simulink model "Trim_Model"  (R2012b)
settings: Solver=ode23tb  StartTime=0.0  StopTime=inf  FixedStep=0.001  MaxStep=0.01  RelTol=1e-5
values from neighbouring files (symbols this model uses):
  a = 2.1117    [SetupComplete.m]
  A_x = 0.015    [SetupComplete.m]
  A_y = A_x    (= 0.015)    [SetupComplete.m]
  A_z = 0.16    [SetupComplete.m]
  C_d0 = 0.00209    [SetupComplete.m]
  C_x = 1.2    [SetupComplete.m]
  C_y = C_x    (= 1.2)    [SetupComplete.m]
  C_z = 2.2    [SetupComplete.m]
  CG_0 = [0,0,0.02]'    [SetupComplete.m]
  h = 0.08    [SetupComplete.m]
  h_FA = 0.02    [SetupComplete.m]
  h_M = 0.064    [SetupComplete.m]
  I_BAC_0 = [ Ix,0,Ixz;0,Iy,0;Ixz,0,Iz]    [SetupComplete.m]
  I_prop = 1/4*M_eq*R^2*diag([1,1,2])    [SetupComplete.m]
  I_tube = [1/2*M_tube*R_tube_eq^2,0,  0  ;           0 ,1/3*M_tube*l_arm^2,0;             0  ,0,1/3*M_tube*l_arm^2]    [SetupComplete.m]
  Initial_Omegas = [1;1;1]*Omega_hover    [Run3Copter.m]
  Initial_Torques = [1;1;1]*Torque_hover    [Run3Copter.m]
  J_FA = I_prop(1,1) + m_prop*h^2  + m_FA*h_FA^2 + m_M*h_M^2    [SetupComplete.m]
  J_T = J_m+1/2*M_eq*R^2    (= 2.000642e-05)    [SetupComplete.m]
  l = 0.345    [SetupComplete.m]
  l_arm = 0.264    [SetupComplete.m]
  m = 3.51    [SetupComplete.m]
  m_0 = 2.61    [SetupComplete.m]
  m_FA = 0.02    [SetupComplete.m]
  m_M = 0.300    (= 0.3)    [SetupComplete.m]
  m_prop = 0.02    [SetupComplete.m]
  Omega_hover = 570    [SetupComplete.m]
  R = 0.1778    [SetupComplete.m]
  rho = 1.15    [SetupComplete.m]
  Rotation_sign = [ 1,-1,-1]    [SetupComplete.m]
  sigma = b*c/(pi*R)    (= 0.107416159567)    [SetupComplete.m]
  Tau_motors = 0.06    [SetupComplete.m]
  theta_0 = 0.38397    [SetupComplete.m]
  theta_1 = -0.2967    [SetupComplete.m]
  Throttle_Hover = X(1)/16    [SetupComplete.m]
  v_i0 = sqrt( 1/3*m*g/(2*rho*pi*R^2)  )    [SetupComplete.m]
undefined symbols (not defined in the file or in its folder): Omega_TTO, Throtle_TTO, Torque_TTO, v_i_adim, Vx_adim, Vz_adim
libraries: vrlib x15, dspmtrx3 x11, simulink_extras x4, aerolibtransform2 x1
(part 2 of 2)

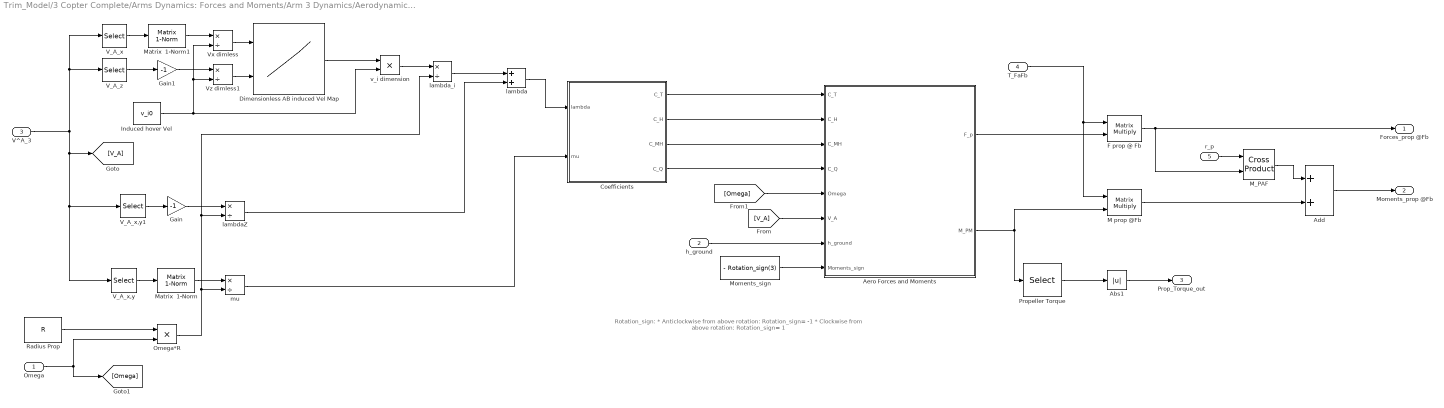
== system Trim_Model/3 Copter Complete/Arms Dynamics: Forces and Moments/Arm 3 Dynamics/Aerodynamics Propeller ==
  note: Rotation_sign:
      |
      | * Anticlockwise from above rotation: Rotation_sign= -1
      | * Clockwise from above rotation: Rotation_sign= 1
  Omega : Inport
  h_ground : Inport  Port=2
  "V^A_3 " : Inport  Port=3
  T_FaFb : Inport  Port=4
  r_p : Inport  Port=5
  Abs1 : Abs
  Add : Sum
  Aero Forces and Moments : MATLAB Function  TreatAsAtomicUnit=on
  Coefficients : MATLAB Function  TreatAsAtomicUnit=on
  Dimensionless AB induced Vel Map : Lookup_n-D  BreakpointsForDimension1=Vx_adim  BreakpointsForDimension2=Vz_adim  BreakpointsForDimension3=[5, 7]  Table=v_i_adim  RndMeth=Simplest  InputSameDT=on
  F prop @ Fb : Product  Multiplication=Matrix(*)
  Gain : Gain  Gain=-1
  Gain1 : Gain  Gain=-1
  Induced hover Vel : Constant  Value=v_i0
  M prop @Fb : Product  Multiplication=Matrix(*)
  M_PAF : vrlib/Utilities/Cross Product
  Matrix  1-Norm : dspmtrx3/Matrix  1-Norm  outputDataTypeStr=Inherit: Same as accumulator  outputLastDataTypeStr=Inherit: Same as accumulator  outputMin=[]  outputMax=[]  roundingMode=Floor  overflowMode=off
  Matrix  1-Norm1 : dspmtrx3/Matrix  1-Norm  outputDataTypeStr=Inherit: Same as accumulator  outputLastDataTypeStr=Inherit: Same as accumulator  outputMin=[]  outputMax=[]  roundingMode=Floor  overflowMode=off
  Moments_sign : Constant  Value=- Rotation_sign(3)
  Omega*R : Product  Inputs=**
  Propeller Torque : Selector  InputPortWidth=3  IndexOptions=Index vector (dialog)  Indices=3  OutputSizes=1
  Radius Prop : Constant  Value=R
  V_A_x : Selector  InputPortWidth=3  IndexOptions=Index vector (dialog)  Indices=[1 2]  OutputSizes=1
  V_A_x,y : Selector  InputPortWidth=3  IndexOptions=Index vector (dialog)  Indices=[1 2]  OutputSizes=1
  V_A_x,y1 : Selector  InputPortWidth=3  IndexOptions=Index vector (dialog)  Indices=[3]  OutputSizes=1
  V_A_z : Selector  InputPortWidth=3  IndexOptions=Index vector (dialog)  Indices=3  OutputSizes=1
  Vx dimless : Product  Inputs=*/
  Vz dimless1 : Product  Inputs=*/
  lambda : Sum
  lambdaZ : Product  Inputs=*/
  lambda_i : Product  Inputs=*/
  mu : Product  Inputs=*/
  v_i dimension : Product  Inputs=**
  Forces_prop @Fb : Outport
  Moments_prop @Fb : Outport  Port=2
  Prop_Torque_out : Outport  Port=3
  wires:
  Radius Prop/1 -> Omega*R/1
  Omega/1 -> Omega*R/2, [Omega]
  V_A_x,y/1 -> Matrix  1-Norm/1
  Matrix  1-Norm/1 -> mu/1
  Omega*R/1 -> mu/2, lambdaZ/2, lambda_i/2
  Vx dimless/1 -> Dimensionless AB induced Vel Map/1
  Vz dimless1/1 -> Dimensionless AB induced Vel Map/2
  Dimensionless AB induced Vel Map/1 -> v_i dimension/1
  v_i dimension/1 -> lambda_i/1
  V_A_x,y1/1 -> Gain/1
  Gain/1 -> lambdaZ/1
  lambda_i/1 -> lambda/1
  lambdaZ/1 -> lambda/2
  lambda/1 -> Coefficients/1(lambda)
  mu/1 -> Coefficients/2(mu)
  Coefficients/1(C_T) -> Aero Forces and Moments/1(C_T)
  Coefficients/2(C_H) -> Aero Forces and Moments/2(C_H)
  Coefficients/3(C_MH) -> Aero Forces and Moments/3(C_MH)
  Coefficients/4(C_Q) -> Aero Forces and Moments/4(C_Q)
  [V_A] -> Aero Forces and Moments/6(V_A)
  [Omega] -> Aero Forces and Moments/5(Omega)
  Aero Forces and Moments/2(M_PM) -> Propeller Torque/1, M prop @Fb/2
  Add/1 -> Moments_prop @Fb/1
  h_ground/1 -> Aero Forces and Moments/7(h_ground)
  Moments_sign/1 -> Aero Forces and Moments/8(Moments_sign)
  Propeller Torque/1 -> Abs1/1
  T_FaFb/1 -> M prop @Fb/1, F prop @ Fb/1
  Aero Forces and Moments/1(F_p) -> F prop @ Fb/2
  F prop @ Fb/1 -> M_PAF/2, Forces_prop @Fb/1
  r_p/1 -> M_PAF/1
  M_PAF/1 -> Add/1
  M prop @Fb/1 -> Add/2
  Abs1/1 -> Prop_Torque_out/1
  "V^A_3 "/1 -> [V_A], V_A_x,y1/1, V_A_x,y/1, V_A_z/1, V_A_x/1
  V_A_x/1 -> Matrix  1-Norm1/1
  V_A_z/1 -> Gain1/1
  Induced hover Vel/1 -> Vz dimless1/2, Vx dimless/2, v_i dimension/2
  Gain1/1 -> Vz dimless1/1
  Matrix  1-Norm1/1 -> Vx dimless/1

== system Trim_Model/3 Copter Complete/Arms Dynamics: Forces and Moments/Arm 3 Dynamics/Arms Kinematics ==
  note: Input angles in rads
      |
      | 1. eta_3 (rad)  (Pan arm 3)
      | 2. gamma_3 (rad)  (Tilt arm 3)
  Angles (rad) : Inport
  Angles_dot (rad/s) : Inport  Port=2
  Add : Sum
  Add3 : Sum
  Bus Creator : BusCreator  Inputs=2
  Cross Product : vrlib/Utilities/Cross Product
  DCM Arm 3 : MATLAB Function  TreatAsAtomicUnit=on
  Demux : Demux  Outputs=2
  Demux3 : Demux  Outputs=2
  Fa->Fb : Product  Multiplication=Matrix(*)
  Gain6 : Gain  Gain=[0;1;0]
  Gain7 : Gain  Gain=[0;0;-1]
  Gain8 : Gain  Gain=[-1/2;-sqrt(3)/2;0]
  Gain9 : Gain  Gain=[1;0;0]
  Matrix Multiply : Product  Multiplication=Matrix(*)
  Transpose : dspmtrx3/Transpose  Hermitian=off  overflowFlag=off
  h arm : Constant  Value=h
  length arm : Constant  Value=l
  r_p3 (m) : Outport
  r_p3_dot (m/s) : Outport  Port=2
  Arm DCMs : Outport  Port=3
  omega^3_Ab (rad/s) : Outport  Port=4
  wires:
  DCM Arm 3/1(T_Fb_FA) -> Transpose/1, Bus Creator/1  "T^3_Fb,FA"
  Bus Creator/1 -> Arm DCMs/1
  Transpose/1 -> [T3_F_aFb], Bus Creator/2  "T^3_F_a,Fb"
  Angles (rad)/1 -> Demux/1
  Demux/1 -> DCM Arm 3/1(eta_3)
  Demux/2 -> DCM Arm 3/2(gamma_3)
  Angles_dot (rad/s)/1 -> Demux3/1
  Demux3/2 -> Gain9/1  "gamma_dot_3"
  Demux3/1 -> Gain6/1  "eta_dot_3"
  Gain9/1 -> Matrix Multiply/2
  [T3_F_aFb] -> Matrix Multiply/1
  Matrix Multiply/1 -> Add/2
  Gain6/1 -> Add/1
  Add/1 -> Cross Product/1, omega^3_Ab (rad/s)/1  "omega^3_Ab"
  Add3/1 -> r_p3 (m)/1  "r_p3 (m)"
  length arm/1 -> Gain8/1
  h arm/1 -> Gain7/1
  Gain7/1 -> Fa->Fb/2
  [T3_F_aFb] -> Fa->Fb/1
  Gain8/1 -> Add3/1
  Fa->Fb/1 -> Cross Product/2, Add3/2
  Cross Product/1 -> r_p3_dot (m/s)/1

== system Trim_Model/3 Copter Complete/Arms Dynamics: Forces and Moments/Arm 3 Dynamics/ESC-MOTOR dynamics1 ==
  note: 1) Only subsystems can be added as variant choices at this level
      | 2) Blocks cannot be connected at this level as connectivity is
      | automatically determined at simulation, based on the active variant
  Throttle : Inport
  Omega : Inport  Port=2
  Initial Omega : Inport  Port=3
  Prop Torque : Inport  Port=4
  ESC+Motor Dynamcis COMPLETED : Subsystem  TreatAsAtomicUnit=on  VariantObject=Variant_completed
  ESC+Motor Dynamcis SYMPLIFIED : Subsystem  TreatAsAtomicUnit=on  VariantObject=Variant_simple
  Omega_out : Outport
  Omega_dot_out : Outport  Port=2

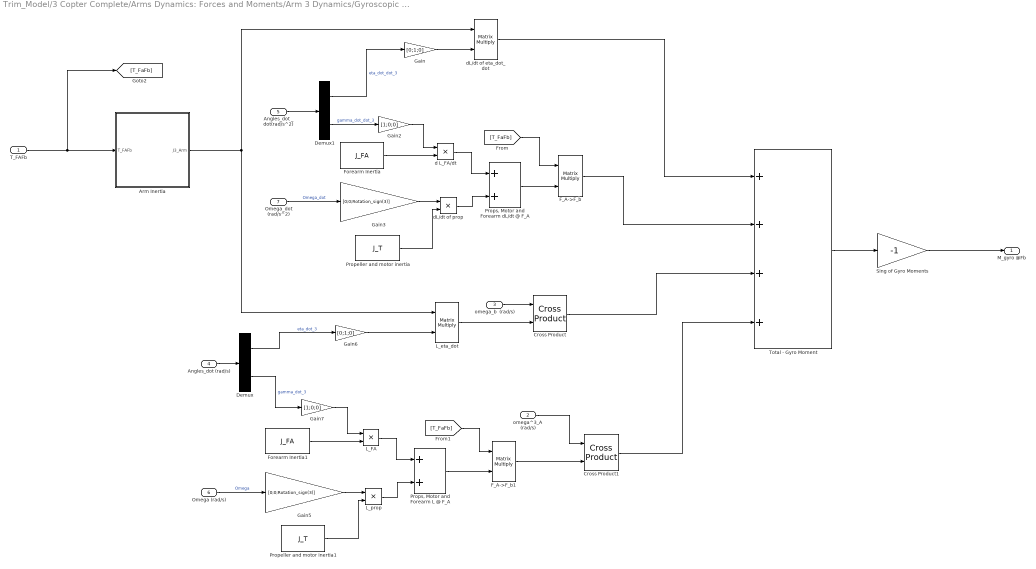
== system Trim_Model/3 Copter Complete/Arms Dynamics: Forces and Moments/Arm 3 Dynamics/Gyroscopic Moments ==
  T_FAFb : Inport
  omega^3_A  (rad/s) : Inport  Port=2
  omega_b  (rad/s) : Inport  Port=3
  Angles_dot (rad/s) : Inport  Port=4
  Angles_dot _dot(rad/s^2) : Inport  Port=5
  Omega (rad/s) : Inport  Port=6
  Omega_dot (rad/s^2) : Inport  Port=7
  Arm Inertia : MATLAB Function  TreatAsAtomicUnit=on
  Cross Product : vrlib/Utilities/Cross Product
  Cross Product1 : vrlib/Utilities/Cross Product
  Demux : Demux  Outputs=2
  Demux1 : Demux  Outputs=2
  F_A->F_b : Product  Multiplication=Matrix(*)
  F_A->F_b1 : Product  Multiplication=Matrix(*)
  Forearm Inertia : Constant  Value=J_FA
  Forearm Inertia1 : Constant  Value=J_FA
  Gain : Gain  Gain=[0;1;0]
  Gain2 : Gain  Gain=[1;0;0]
  Gain3 : Gain  Gain=[0;0;Rotation_sign(3)]
  Gain5 : Gain  Gain=[0;0;Rotation_sign(3)]
  Gain6 : Gain  Gain=[0;1;0]
  Gain7 : Gain  Gain=[1;0;0]
  L_FA : Product  Inputs=**
  L_eta_dot : Product  Multiplication=Matrix(*)
  L_prop : Product  Inputs=**
  Propeller and motor inertia : Constant  Value=J_T
  Propeller and motor inertia1 : Constant  Value=J_T
  "Props, Motor and Forearm L @ F_A" : Sum
  "Props, Motor and Forearm dL/dt @ F_A" : Sum
  Sing of Gyro Moments : Gain  Gain=-1
  Total - Gyro Moment : Sum  Inputs=++++
  d L_FA/dt : Product  Inputs=**
  dL/dt of eta_dot_dot : Product  Multiplication=Matrix(*)
  dL/dt of prop : Product  Inputs=**
  M_gyro @Fb : Outport
  wires:
  T_FAFb/1 -> [T_FaFb], Arm Inertia/1(T_FAFb)
  Angles_dot (rad/s)/1 -> Demux/1
  Angles_dot _dot(rad/s^2)/1 -> Demux1/1
  Demux1/1 -> Gain/1  "eta_dot_dot_3"
  Arm Inertia/1(J3_Arm) -> dL/dt of eta_dot_dot/1, L_eta_dot/1
  Gain/1 -> dL/dt of eta_dot_dot/2
  Gain6/1 -> L_eta_dot/2
  Demux/1 -> Gain6/1  "eta_dot_3"
  L_eta_dot/1 -> Cross Product/2
  omega_b  (rad/s)/1 -> Cross Product/1
  Demux1/2 -> Gain2/1  "gamma_dot_dot_3"
  Gain2/1 -> d L_FA/dt/1
  Forearm Inertia/1 -> d L_FA/dt/2
  Omega_dot (rad/s^2)/1 -> Gain3/1  "Omega_dot"
  Gain3/1 -> dL/dt of prop/1
  Propeller and motor inertia/1 -> dL/dt of prop/2
  d L_FA/dt/1 -> "Props, Motor and Forearm dL/dt @ F_A"/1
  dL/dt of prop/1 -> "Props, Motor and Forearm dL/dt @ F_A"/2
  Demux/2 -> Gain7/1  "gamma_dot_3"
  Gain7/1 -> L_FA/1
  Forearm Inertia1/1 -> L_FA/2
  Gain5/1 -> L_prop/1
  Propeller and motor inertia1/1 -> L_prop/2
  L_FA/1 -> "Props, Motor and Forearm L @ F_A"/1
  L_prop/1 -> "Props, Motor and Forearm L @ F_A"/2
  Omega (rad/s)/1 -> Gain5/1  "Omega"
  "Props, Motor and Forearm dL/dt @ F_A"/1 -> F_A->F_b/2
  F_A->F_b/1 -> Total - Gyro Moment/2
  dL/dt of eta_dot_dot/1 -> Total - Gyro Moment/1
  Cross Product/1 -> Total - Gyro Moment/3
  "Props, Motor and Forearm L @ F_A"/1 -> F_A->F_b1/2
  [T_FaFb] -> F_A->F_b/1
  [T_FaFb] -> F_A->F_b1/1
  F_A->F_b1/1 -> Cross Product1/2
  omega^3_A  (rad/s)/1 -> Cross Product1/1
  Cross Product1/1 -> Total - Gyro Moment/4
  Total - Gyro Moment/1 -> Sing of Gyro Moments/1
  Sing of Gyro Moments/1 -> M_gyro @Fb/1

== system Trim_Model/3 Copter Complete/Arms Dynamics: Forces and Moments/Arm 3 Dynamics/Servos Dynamics ==
  Com Angles (rad) : Inport
  Torques? : Inport  Port=2
  Demux : Demux  Outputs=2
  Derivative : Derivative  CoefficientInTFapproximation=0
  Derivative1 : Derivative  Commented=on  CoefficientInTFapproximation=0
  Derivative2 : Derivative  Commented=on  CoefficientInTFapproximation=0
  Derivative3 : Derivative  Commented=on  CoefficientInTFapproximation=0
  Mux : Mux  Inputs=2
  Mux1 : Mux  Commented=on  Inputs=2
  Mux2 : Mux  Commented=on  Inputs=2
  eta_3 : TransferFcn  Numerator=[1230]  Denominator=[1 50 1230]
  gamma_3 : TransferFcn  Numerator=[1230]  Denominator=[1 50 1230]
  Angles Arms (rad) : Outport
  Angles_dot (rad/s) : Outport  Port=2
  Angles_dot_dot (rad/s^2) : Outport  Port=3
  wires:
  Demux/1 -> eta_3/1
  Demux/2 -> gamma_3/1
  Com Angles (rad)/1 -> Angles Arms (rad)/1, Demux/1
  eta_3/1 -> Derivative/1, Mux/1
  gamma_3/1 -> Mux/2, Derivative1/1
  Mux1/1 -> Angles_dot (rad/s)/1
  Mux2/1 -> Angles_dot_dot (rad/s^2)/1
  Derivative1/1 -> Derivative3/1, Mux1/2
  Derivative2/1 -> Mux2/1
  Derivative3/1 -> Mux2/2
  Derivative/1 -> Mux1/1, Derivative2/1

== system Trim_Model/3 Copter Complete/Arms Dynamics: Forces and Moments/Arm 1 Dynamics/ESC-MOTOR dynamics/ESC+Motor Dynamcis COMPLETED ==
  Throttle : Inport
  Omega : Inport  Port=2
  Initial Omega : Inport  Port=3
  Prop Torque : Inport  Port=4
  2-D Torque-Throttle-Omega Map : Lookup_n-D  BreakpointsForDimension1=Torque_TTO(:,1)  BreakpointsForDimension2=Throtle_TTO(1,:)  Table=Omega_TTO  ExtrapMethod=Clip  DiagnosticForOutOfRangeInput=Warning  RemoveProtectionInput=on  RndMeth=Simplest  InputSameDT=on
  Add : Sum  Inputs=+-
  Add1 : Sum
  Display : Display
  Divide : Product  Inputs=*/
  Divide1 : Product  Inputs=**
  Inerti of prop+motor : Constant  Value=J_T
  Integrator : Integrator  Commented=on  InitialConditionSource=external
  Manual Switch : ManualSwitch
  Memory4 : Memory
  Time constant motors : Constant  Value=Tau_motors
  null : Constant  Value=0
  Omega_out : Outport
  Omega_dot_out : Outport  Port=2
  wires:
  Prop Torque/1 -> Add1/1
  2-D Torque-Throttle-Omega Map/1 -> Display/1, Omega_out/1, Add/1
  Omega/1 -> Add/2
  Add/1 -> Divide/1
  Time constant motors/1 -> Divide/2
  Initial Omega/1 -> Integrator/2
  Manual Switch/1 -> Add1/2
  Inerti of prop+motor/1 -> Divide1/1
  Divide1/1 -> Manual Switch/2
  null/1 -> Manual Switch/1
  Throttle/1 -> 2-D Torque-Throttle-Omega Map/2
  Add1/1 -> 2-D Torque-Throttle-Omega Map/1
  Divide/1 -> Omega_dot_out/1, Memory4/1, Integrator/1
  Memory4/1 -> Divide1/2

== system Trim_Model/3 Copter Complete/Arms Dynamics: Forces and Moments/Arm 1 Dynamics/ESC-MOTOR dynamics/ESC+Motor Dynamcis SYMPLIFIED ==
  Throttle : Inport
  Omega : Inport  Port=2
  Initial Omega : Inport  Port=3
  Prop Torque : Inport  Port=4
  Add : Sum  Inputs=-+
  Add1 : Sum  Inputs=+-
  Add2 : Sum
  Example Motor TF : TransferFcn  Numerator=9  Denominator=[0.16 1]
  Example Motor TF1 : TransferFcn  Numerator=[9,0]  Denominator=[0.16 1]
  Omega_hover : Constant  Value=Omega_hover
  Terminator : Terminator
  Terminator1 : Terminator
  Throttle_Hover : Constant  Value=Throttle_Hover
  Omega_out : Outport
  Omega_dot_out : Outport  Port=2
  wires:
  Add2/1 -> Omega_out/1
  Example Motor TF1/1 -> Omega_dot_out/1
  Add/1 -> Example Motor TF/1, Example Motor TF1/1
  Throttle_Hover/1 -> Add/1
  Throttle/1 -> Add/2
  Omega/1 -> Add1/1
  Omega_hover/1 -> Add1/2
  Example Motor TF/1 -> Add2/1
  Add1/1 -> Add2/2
  Initial Omega/1 -> Terminator/1
  Prop Torque/1 -> Terminator1/1

== system Trim_Model/3 Copter Complete/Arms Dynamics: Forces and Moments/Arm 2 Dynamics/ESC-MOTOR dynamics1/ESC+Motor Dynamcis COMPLETED ==
  Throttle : Inport
  Omega : Inport  Port=2
  Initial Omega : Inport  Port=3
  Prop Torque : Inport  Port=4
  2-D Torque-Throttle-Omega Map : Lookup_n-D  BreakpointsForDimension1=Torque_TTO(:,1)  BreakpointsForDimension2=Throtle_TTO(1,:)  Table=Omega_TTO  ExtrapMethod=Clip  DiagnosticForOutOfRangeInput=Warning  RemoveProtectionInput=on  RndMeth=Simplest  InputSameDT=on
  Add : Sum  Inputs=+-
  Add1 : Sum
  Display : Display
  Display1 : Display
  Display2 : Display
  Divide : Product  Inputs=*/
  Divide1 : Product  Inputs=**
  Inerti of prop+motor : Constant  Value=J_T
  Integrator : Integrator  Commented=on  InitialConditionSource=external
  Manual Switch : ManualSwitch
  Time constant motors : Constant  Value=Tau_motors
  Torque : Scope
      settings: TimeRange=10  YMin=0.16  YMax=0.31  SaveName=ScopeData3
  null : Constant  Value=0
  omega : Scope
      settings: TimeRange=10  YMin=540  YMax=615  SaveName=ScopeData5
  Omega_out : Outport
  Omega_dot_out : Outport  Port=2
  wires:
  Throttle/1 -> Display2/1, 2-D Torque-Throttle-Omega Map/2
  null/1 -> Manual Switch/1
  Divide1/1 -> Manual Switch/2
  Inerti of prop+motor/1 -> Divide1/1
  Manual Switch/1 -> Add1/2
  Add1/1 -> Display1/1, Torque/1, 2-D Torque-Throttle-Omega Map/1
  2-D Torque-Throttle-Omega Map/1 -> Omega_out/1, Add/1, omega/1, Display/1
  Divide/1 -> Omega_dot_out/1, Integrator/1, Divide1/2
  Initial Omega/1 -> Integrator/2
  Time constant motors/1 -> Divide/2
  Add/1 -> Divide/1
  Omega/1 -> Add/2
  Prop Torque/1 -> Add1/1

== system Trim_Model/3 Copter Complete/Arms Dynamics: Forces and Moments/Arm 2 Dynamics/ESC-MOTOR dynamics1/ESC+Motor Dynamcis SYMPLIFIED ==
  Throttle : Inport
  Omega : Inport  Port=2
  Initial Omega : Inport  Port=3
  Prop Torque : Inport  Port=4
  Add : Sum  Inputs=-+
  Add1 : Sum  Inputs=+-
  Add2 : Sum
  Example Motor TF : TransferFcn  Numerator=9  Denominator=[0.16 1]
  Example Motor TF1 : TransferFcn  Numerator=[9,0]  Denominator=[0.16 1]
  Omega_hover : Constant  Value=Omega_hover
  Terminator : Terminator
  Terminator1 : Terminator
  Throttle_Hover : Constant  Value=Throttle_Hover
  Omega_out : Outport
  Omega_dot_out : Outport  Port=2
  wires:
  Add2/1 -> Omega_out/1
  Example Motor TF1/1 -> Omega_dot_out/1
  Add/1 -> Example Motor TF/1, Example Motor TF1/1
  Throttle_Hover/1 -> Add/1
  Throttle/1 -> Add/2
  Omega/1 -> Add1/1
  Omega_hover/1 -> Add1/2
  Example Motor TF/1 -> Add2/1
  Add1/1 -> Add2/2
  Initial Omega/1 -> Terminator/1
  Prop Torque/1 -> Terminator1/1

== system Trim_Model/3 Copter Complete/Arms Dynamics: Forces and Moments/Arm 3 Dynamics/ESC-MOTOR dynamics1/ESC+Motor Dynamcis COMPLETED ==
  Throttle : Inport
  Omega : Inport  Port=2
  Initial Omega : Inport  Port=3
  Prop Torque : Inport  Port=4
  2-D Torque-Throttle-Omega Map : Lookup_n-D  BreakpointsForDimension1=Torque_TTO(:,1)  BreakpointsForDimension2=Throtle_TTO(1,:)  Table=Omega_TTO  ExtrapMethod=Clip  DiagnosticForOutOfRangeInput=Warning  RemoveProtectionInput=on  RndMeth=Simplest  InputSameDT=on
  Add : Sum  Inputs=+-
  Add1 : Sum
  Divide : Product  Inputs=*/
  Divide1 : Product  Inputs=**
  Inerti of prop+motor : Constant  Value=J_T
  Integrator : Integrator  Commented=on  InitialConditionSource=external
  Manual Switch : ManualSwitch
  Time constant motors : Constant  Value=Tau_motors
  null : Constant  Value=0
  Omega_out : Outport
  Omega_dot_out : Outport  Port=2
  wires:
  Throttle/1 -> 2-D Torque-Throttle-Omega Map/2
  null/1 -> Manual Switch/1
  Divide1/1 -> Manual Switch/2
  Inerti of prop+motor/1 -> Divide1/1
  Manual Switch/1 -> Add1/2
  Add1/1 -> 2-D Torque-Throttle-Omega Map/1
  2-D Torque-Throttle-Omega Map/1 -> Omega_out/1, Add/1
  Divide/1 -> Omega_dot_out/1, Integrator/1, Divide1/2
  Initial Omega/1 -> Integrator/2
  Time constant motors/1 -> Divide/2
  Add/1 -> Divide/1
  Omega/1 -> Add/2
  Prop Torque/1 -> Add1/1

== system Trim_Model/3 Copter Complete/Arms Dynamics: Forces and Moments/Arm 3 Dynamics/ESC-MOTOR dynamics1/ESC+Motor Dynamcis SYMPLIFIED ==
  Throttle : Inport
  Omega : Inport  Port=2
  Initial Omega : Inport  Port=3
  Prop Torque : Inport  Port=4
  Add : Sum  Inputs=-+
  Add1 : Sum  Inputs=+-
  Add2 : Sum
  Example Motor TF : TransferFcn  Numerator=9  Denominator=[0.16 1]
  Example Motor TF1 : TransferFcn  Numerator=[9,0]  Denominator=[0.16 1]
  Omega_hover : Constant  Value=Omega_hover
  Terminator : Terminator
  Terminator1 : Terminator
  Throttle_Hover : Constant  Value=Throttle_Hover
  Omega_out : Outport
  Omega_dot_out : Outport  Port=2
  wires:
  Prop Torque/1 -> Terminator1/1
  Initial Omega/1 -> Terminator/1
  Add1/1 -> Add2/2
  Example Motor TF/1 -> Add2/1
  Omega_hover/1 -> Add1/2
  Omega/1 -> Add1/1
  Throttle/1 -> Add/2
  Throttle_Hover/1 -> Add/1
  Add/1 -> Example Motor TF1/1, Example Motor TF/1
  Example Motor TF1/1 -> Omega_dot_out/1
  Add2/1 -> Omega_out/1

== matlab function Trim_Model/3 Copter Complete/Gravity Force and Moment ==
  data: q input; F_g_b output; M_g_b output; mass input; CG input; g parameter
function [F_g_b,M_g_b]   = Grav_Forces_and_Mom( q,mass,CG, g)

Prod=HamiltonProduct([q(1);-q(2);-q(3);-q(4)],HamiltonProduct([0;0;0;mass*g],[q(1);q(2);q(3);q(4)]) ); % q* . g .q

F_g_b= Prod(2:4);
M_g_b=cross(CG,F_g_b);
end

== matlab function Trim_Model/3 Copter Complete/Aerodynamics body Force and Moment1 ==
  data: V_b input; F_a_b output; M_a_b output; rho parameter; C_x parameter; C_y parameter; C_z parameter; A_x parameter; A_y parameter; A_z parameter
function [F_a_b,M_a_b]   = Aero_body_Forces_and_Mom( V_b, rho,C_x,C_y,C_z,A_x,A_y,A_z)


F_a_b=1/2*rho*(V_b*V_b')*[C_x*A_x;C_y*A_y;C_z*A_z].*( - V_b./(norm(V_b)+eps) );
M_a_b=[0;0;0];
end

== matlab function Trim_Model/3 Copter Complete/Arms Dynamics: Forces and Moments/Arm 1 Dynamics/Aerodynamics Propeller/Coefficients ==
  data: lambda input; C_T output; mu input; C_H output; C_MH output; C_Q output; sigma parameter; C_d0 parameter; a parameter; theta_0 parameter; theta_1 parameter
function [C_T,C_H,C_MH,C_Q] = Aero_coeff(lambda,mu, sigma, C_d0, a, theta_0, theta_1)

C_T = sigma*a/4*(theta_0*(2/3+mu^2) +theta_1/2*(1+mu^2) +  lambda );
C_Q =    +sigma*a/4*( 2/3*theta_0 + lambda + theta_1/2)*lambda + sigma*C_d0/8*(1+mu^2);   % Always positive!!!


C_H= -sigma*a/4*mu*lambda*(theta_0+theta_1/2) + sigma*C_d0/4*mu; 
C_MH= sigma*a/4*( 2/3*theta_0*mu+1/2*lambda*mu+theta_1*mu/2  );

== matlab function Trim_Model/3 Copter Complete/Arms Dynamics: Forces and Moments/Arm 1 Dynamics/Aerodynamics Propeller/Aero Forces and Moments ==
  data: C_T input; C_H input; C_MH input; C_Q input; F_p output; M_PM output; Omega input; V_A input; h_ground input; Moments_sign input; R parameter; rho parameter
function [F_p,M_PM] = Aero_Forces_and_Moments(C_T,C_H,C_MH,C_Q,Omega,V_A,h_ground,Moments_sign, R, rho)



if V_A(1)==0 && V_A(2)==0
    H=[0;0];
else
    H=C_H*(-[V_A(1);V_A(2)])./norm([V_A(1);V_A(2)]);
end
%     C_T

T_temp=1/(1-R^2/(16*h_ground^2))*C_T;

F_p =   rho*pi*R^2*(Omega*R)^2*  [  H ; -T_temp ];
% pause

% Moments
% %     Moments_sign=1; % Anticlockwise from above
% %     Moments_sign=-1; % Clockwise from above 2y 4
if V_A(1)==0 && V_A(2)==0
    Mh=[0;0];
else
    Mh=Moments_sign*C_MH*(-[V_A(1);V_A(2)])./norm([V_A(1);V_A(2)]);% Note!!!! Signum of C_Mh depends on the spinning direction???
end

M_PM = rho*pi*R^3*(Omega*R)^2* [  Mh  ;  Moments_sign*C_Q ] ;

== matlab function Trim_Model/3 Copter Complete/Arms Dynamics: Forces and Moments/Arm 1 Dynamics/Arms Kinematics/DCM Arm 1 ==
  data: eta_1 input; T_Fb_FA output; gamma_1 input
function T_Fb_FA = DCM_Arm_1(eta_1, gamma_1)

T_Fb_FA = [ cos(gamma_1), sin(eta_1)*sin(gamma_1), -cos(eta_1)*sin(gamma_1);...
            0,cos(eta_1),sin(eta_1);...
            sin(gamma_1),-cos(gamma_1)*sin(eta_1),cos(gamma_1)*cos(eta_1) ];

== matlab function Trim_Model/3 Copter Complete/Arms Dynamics: Forces and Moments/Arm 1 Dynamics/Gyroscopic Moments/Arm Inertia ==
  data: T_FAFb input; J1_Arm output; I_tube parameter; I_prop parameter; l_arm parameter; h_FA parameter; h_M parameter; h parameter; m_FA parameter; m_M parameter; m_prop parameter
function J1_Arm  = Arm1_inertia(T_FAFb, I_tube, I_prop, l_arm, h_FA, h_M, h, m_FA, m_M, m_prop)


r_FAO=[l_arm;0;0]+T_FAFb*[0;0;-h_FA];
r_MO=[l_arm;0;0]+T_FAFb*[0;0;-h_M];
r_po=[l_arm;0;0]+T_FAFb*[0;0;-h];

I_FA = m_FA*[ r_FAO(2)^2+r_FAO(3)^2,r_FAO(1)*r_FAO(2),r_FAO(1)*r_FAO(3);...
            r_FAO(1)*r_FAO(2), r_FAO(1)^2+r_FAO(3)^2, r_FAO(2)*r_FAO(3);...
            r_FAO(1)*r_FAO(3),r_FAO(2)*r_FAO(3), r_FAO(1)^2+r_FAO(2)^2];
I_M = m_M*[ r_MO(2)^2+r_MO(3)^2,r_MO(1)*r_MO(2),r_MO(1)*r_MO(3);...
            r_MO(1)*r_MO(2), r_MO(1)^2+r_MO(3)^2, r_MO(2)*r_MO(3);...
            r_MO(1)*r_MO(3),r_MO(2)*r_MO(3), r_MO(1)^2+r_MO(2)^2];
I_stiner = m_prop*[ r_po(2)^2+r_po(3)^2,r_po(1)*r_po(2),r_po(1)*r_po(3);...
            r_po(1)*r_po(2), r_po(1)^2+r_po(3)^2, r_po(2)*r_po(3);...
            r_po(1)*r_po(3),r_po(2)*r_po(3), r_po(1)^2+r_po(2)^2];

J1_Arm = T_FAFb*I_prop*T_FAFb'+ I_tube +I_FA+I_M+I_stiner;

== matlab function Trim_Model/3 Copter Complete/Mass Properties/Arm Inertia ==
  data: T1_FAFb input; T2_FAFb input; T3_FAFb input; I_M output; l parameter; h_M parameter; m_M parameter; r1_M output; r2_M output; r3_M output
function [I_M,r1_M,r2_M,r3_M]  = Arm1_inertia(T1_FAFb,T2_FAFb,T3_FAFb, l, h_M, m_M)


r1_M=[l;0;0]+T1_FAFb*[0;0;-h_M];
r2_M=[-1/2*l;sqrt(3)/2*l;0]+T2_FAFb*[0;0;-h_M];
r3_M=[-1/2*l;-sqrt(3)/2*l;0]+T3_FAFb*[0;0;-h_M];


I_M1 = m_M*[ r1_M(2)^2+r1_M(3)^2,r1_M(1)*r1_M(2),r1_M(1)*r1_M(3);...
            r1_M(1)*r1_M(2), r1_M(1)^2+r1_M(3)^2, r1_M(2)*r1_M(3);...
            r1_M(1)*r1_M(3),r1_M(2)*r1_M(3), r1_M(1)^2+r1_M(2)^2];
I_M2 = m_M*[ r2_M(2)^2+r2_M(3)^2,r2_M(1)*r2_M(2),r2_M(1)*r2_M(3);...
            r2_M(1)*r2_M(2), r2_M(1)^2+r2_M(3)^2, r2_M(2)*r2_M(3);...
            r2_M(1)*r2_M(3),r2_M(2)*r2_M(3), r2_M(1)^2+r2_M(2)^2];
I_M3 = m_M*[ r3_M(2)^2+r3_M(3)^2,r3_M(1)*r3_M(2),r3_M(1)*r3_M(3);...
            r3_M(1)*r3_M(2), r3_M(1)^2+r3_M(3)^2, r3_M(2)*r3_M(3);...
            r3_M(1)*r3_M(3),r3_M(2)*r3_M(3), r3_M(1)^2+r3_M(2)^2];

I_M = I_M1+I_M2+I_M3;

== matlab function Trim_Model/3 Copter Complete/Arms Dynamics: Forces and Moments/Arm 2 Dynamics/Aerodynamics Propeller/Aero Forces and Moments ==
  data: C_T input; C_H input; C_MH input; C_Q input; F_p output; M_PM output; Omega input; V_A input; h_ground input; Moments_sign input; R parameter; rho parameter
function [F_p,M_PM] = Aero_Forces_and_Moments(C_T,C_H,C_MH,C_Q,Omega,V_A,h_ground,Moments_sign, R, rho)



if V_A(1)==0 && V_A(2)==0
    H=[0;0];
else
    H=C_H*(-[V_A(1);V_A(2)])./norm([V_A(1);V_A(2)]);
end
%     C_T

T_temp=1/(1-R^2/(16*h_ground^2))*C_T;

F_p =   rho*pi*R^2*(Omega*R)^2*  [  H ; -T_temp ];
% pause

% Moments
% %     Moments_sign=1; % Anticlockwise from above
% %     Moments_sign=-1; % Clockwise from above 2y 4
if V_A(1)==0 && V_A(2)==0
    Mh=[0;0];
else
    Mh=Moments_sign*C_MH*(-[V_A(1);V_A(2)])./norm([V_A(1);V_A(2)]);% Note!!!! Signum of C_Mh depends on the spinning direction???
end

M_PM = rho*pi*R^3*(Omega*R)^2* [  Mh  ;  Moments_sign*C_Q ] ;

== matlab function Trim_Model/3 Copter Complete/Arms Dynamics: Forces and Moments/Arm 3 Dynamics/Aerodynamics Propeller/Aero Forces and Moments ==
  data: C_T input; C_H input; C_MH input; C_Q input; F_p output; M_PM output; Omega input; V_A input; h_ground input; Moments_sign input; R parameter; rho parameter
function [F_p,M_PM] = Aero_Forces_and_Moments(C_T,C_H,C_MH,C_Q,Omega,V_A,h_ground,Moments_sign, R, rho)



if V_A(1)==0 && V_A(2)==0
    H=[0;0];
else
    H=C_H*(-[V_A(1);V_A(2)])./norm([V_A(1);V_A(2)]);
end
%     C_T

T_temp=1/(1-R^2/(16*h_ground^2))*C_T;

F_p =   rho*pi*R^2*(Omega*R)^2*  [  H ; -T_temp ];
% pause

% Moments
% %     Moments_sign=1; % Anticlockwise from above
% %     Moments_sign=-1; % Clockwise from above 2y 4
if V_A(1)==0 && V_A(2)==0
    Mh=[0;0];
else
    Mh=Moments_sign*C_MH*(-[V_A(1);V_A(2)])./norm([V_A(1);V_A(2)]);% Note!!!! Signum of C_Mh depends on the spinning direction???
end

M_PM = rho*pi*R^3*(Omega*R)^2* [  Mh  ;  Moments_sign*C_Q ] ;

== matlab function Trim_Model/3 Copter Complete/SVFI_to_SVFb ==
  data: X_e input; V_e input; X_e_out output; V_b output; omega_b output; Euler_Ang input; Euler_Ang_Dot input; q output
function [X_e_out,V_b, omega_b ,q]=SVFI_to_SVFb(X_e,V_e, Euler_Ang,Euler_Ang_Dot)

xp=V_e(1);
yp=V_e(2);
zp=V_e(3);

phi=Euler_Ang(1);
theta=Euler_Ang(2);
psi=Euler_Ang(3);
phip=Euler_Ang_Dot(1);
thetap=Euler_Ang_Dot(2);
psip=Euler_Ang_Dot(3);

%%
X_e_out=X_e;

q = QuaternionfromEuler(phi,theta,psi); 



HamOut=HamiltonProduct([q(1);-q(2);-q(3);-q(4)],HamiltonProduct([0;xp;yp;zp],[q(1);q(2);q(3);q(4)]) );% q* . v . q
V_b=HamOut(2:4);

omega_b=[phip-psip*sin(theta)  ;
         thetap*cos(phi)+psip*cos(theta)*sin(phi);
            -thetap*sin(phi)+psip*cos(theta)*cos(phi)  ];% Ya que es solo una operacion aislada utilizaremos la ecuaciones con rel trigonometricas
end
function [q]=QuaternionfromEuler(phi,theta,psi)
% options=optimset('MaxFunEvals',3000);
% q=fsolve(@QUATERNIONEULER,[0.6,0.4,0.5,0.4]); % Hay que acertar con los angulos poniendo diferentes valores iniciales del quaternion
%     function F=QUATERNIONEULER(q)
%         F=[ tan(phi)-(2*q(3)*q(4)-2*q(1)*q(2))/(2*q(1)^2+2*q(4)^2-1)  ;
%             sin(-theta)-2*q(2)*q(4)-2*q(1)*q(3);
%             tan(psi)-(2*q(2)*q(3)-2*q(1)*q(4))/(2*q(1)^2+2*q(2)^2-1);
%             q(1)^2+q(2)^2+q(3)^2+q(4)^2-1];
%     end  % Este algoritmo da q* !!!!!

q=[ cos(psi/2)*cos(theta/2)*cos(phi/2)+ sin(psi/2)*sin(theta/2)*sin(phi/2) ;
      cos(psi/2)*cos(theta/2)*sin(phi/2)- sin(psi/2)*sin(theta/2)*cos(phi/2) ;
       cos(psi/2)*sin(theta/2)*cos(phi/2)+ sin(psi/2)*cos(theta/2)*sin(phi/2)   ;
        sin(psi/2)*cos(theta/2)*cos(phi/2)- cos(psi/2)*sin(theta/2)*sin(phi/2)      ]; % Esto nos da q !!!
end

== matlab function Trim_Model/3 Copter Complete/Arms Dynamics: Forces and Moments/Arm 2 Dynamics/Aerodynamics Propeller/Coefficients ==
  data: lambda input; C_T output; mu input; C_H output; C_MH output; C_Q output; sigma parameter; C_d0 parameter; a parameter; theta_0 parameter; theta_1 parameter
function [C_T,C_H,C_MH,C_Q] = Aero_coeff(lambda,mu, sigma, C_d0, a, theta_0, theta_1)

C_T = sigma*a/4*(theta_0*(2/3+mu^2) +theta_1/2*(1+mu^2) +  lambda );
C_Q =    +sigma*a/4*( 2/3*theta_0 + lambda + theta_1/2)*lambda + sigma*C_d0/8*(1+mu^2);   % Always positive!!!


C_H= -sigma*a/4*mu*lambda*(theta_0+theta_1/2) + sigma*C_d0/4*mu; 
C_MH= sigma*a/4*( 2/3*theta_0*mu+1/2*lambda*mu+theta_1*mu/2  );

== matlab function Trim_Model/3 Copter Complete/Arms Dynamics: Forces and Moments/Arm 2 Dynamics/Gyroscopic Moments/Arm Inertia ==
  data: T_FAFb input; J2_Arm output; I_tube parameter; I_prop parameter; l_arm parameter; h_FA parameter; h_M parameter; h parameter; m_FA parameter; m_M parameter; m_prop parameter
function J2_Arm  = Arm2_inertia(T_FAFb, I_tube, I_prop, l_arm, h_FA, h_M, h, m_FA, m_M, m_prop)


r_FAO=[0;l_arm;0]+T_FAFb*[0;0;-h_FA];
r_MO=[0;l_arm;0]+T_FAFb*[0;0;-h_M];
r_po=[0;l_arm;0]+T_FAFb*[0;0;-h];

I_FA = m_FA*[ r_FAO(2)^2+r_FAO(3)^2,r_FAO(1)*r_FAO(2),r_FAO(1)*r_FAO(3);...
            r_FAO(1)*r_FAO(2), r_FAO(1)^2+r_FAO(3)^2, r_FAO(2)*r_FAO(3);...
            r_FAO(1)*r_FAO(3),r_FAO(2)*r_FAO(3), r_FAO(1)^2+r_FAO(2)^2];
I_M = m_M*[ r_MO(2)^2+r_MO(3)^2,r_MO(1)*r_MO(2),r_MO(1)*r_MO(3);...
            r_MO(1)*r_MO(2), r_MO(1)^2+r_MO(3)^2, r_MO(2)*r_MO(3);...
            r_MO(1)*r_MO(3),r_MO(2)*r_MO(3), r_MO(1)^2+r_MO(2)^2];
I_stiner = m_prop*[ r_po(2)^2+r_po(3)^2,r_po(1)*r_po(2),r_po(1)*r_po(3);...
            r_po(1)*r_po(2), r_po(1)^2+r_po(3)^2, r_po(2)*r_po(3);...
            r_po(1)*r_po(3),r_po(2)*r_po(3), r_po(1)^2+r_po(2)^2];

J2_Arm = T_FAFb*I_prop*T_FAFb'+ I_tube +I_FA+I_M+I_stiner;

== matlab function Trim_Model/3 Copter Complete/Arms Dynamics: Forces and Moments/Arm 3 Dynamics/Aerodynamics Propeller/Coefficients ==
  data: lambda input; C_T output; mu input; C_H output; C_MH output; C_Q output; sigma parameter; C_d0 parameter; a parameter; theta_0 parameter; theta_1 parameter
function [C_T,C_H,C_MH,C_Q] = Aero_coeff(lambda,mu, sigma, C_d0, a, theta_0, theta_1)

C_T = sigma*a/4*(theta_0*(2/3+mu^2) +theta_1/2*(1+mu^2) +  lambda );
C_Q =    +sigma*a/4*( 2/3*theta_0 + lambda + theta_1/2)*lambda + sigma*C_d0/8*(1+mu^2);   % Always positive!!!


C_H= -sigma*a/4*mu*lambda*(theta_0+theta_1/2) + sigma*C_d0/4*mu; 
C_MH= sigma*a/4*( 2/3*theta_0*mu+1/2*lambda*mu+theta_1*mu/2  );

== matlab function Trim_Model/3 Copter Complete/Arms Dynamics: Forces and Moments/Arm 3 Dynamics/Gyroscopic Moments/Arm Inertia ==
  data: T_FAFb input; J3_Arm output; I_tube parameter; I_prop parameter; l_arm parameter; h_FA parameter; h_M parameter; h parameter; m_FA parameter; m_M parameter; m_prop parameter
function J3_Arm  = Arm3_inertia(T_FAFb, I_tube, I_prop, l_arm, h_FA, h_M, h, m_FA, m_M, m_prop)


r_FAO=[0;-l_arm;0]+T_FAFb*[0;0;-h_FA];
r_MO=[0;-l_arm;0]+T_FAFb*[0;0;-h_M];
r_po=[0;-l_arm;0]+T_FAFb*[0;0;-h];

I_FA = m_FA*[ r_FAO(2)^2+r_FAO(3)^2,r_FAO(1)*r_FAO(2),r_FAO(1)*r_FAO(3);...
            r_FAO(1)*r_FAO(2), r_FAO(1)^2+r_FAO(3)^2, r_FAO(2)*r_FAO(3);...
            r_FAO(1)*r_FAO(3),r_FAO(2)*r_FAO(3), r_FAO(1)^2+r_FAO(2)^2];
I_M = m_M*[ r_MO(2)^2+r_MO(3)^2,r_MO(1)*r_MO(2),r_MO(1)*r_MO(3);...
            r_MO(1)*r_MO(2), r_MO(1)^2+r_MO(3)^2, r_MO(2)*r_MO(3);...
            r_MO(1)*r_MO(3),r_MO(2)*r_MO(3), r_MO(1)^2+r_MO(2)^2];
I_stiner = m_prop*[ r_po(2)^2+r_po(3)^2,r_po(1)*r_po(2),r_po(1)*r_po(3);...
            r_po(1)*r_po(2), r_po(1)^2+r_po(3)^2, r_po(2)*r_po(3);...
            r_po(1)*r_po(3),r_po(2)*r_po(3), r_po(1)^2+r_po(2)^2];

J3_Arm = T_FAFb*I_prop*T_FAFb'+ I_tube +I_FA+I_M+I_stiner;

== matlab function Trim_Model/3 Copter Complete/Arms Dynamics: Forces and Moments/Arm 3 Dynamics/Arms Kinematics/DCM Arm 3 ==
  data: eta_3 input; T_Fb_FA output; gamma_3 input
function T_Fb_FA = DCM_Arm_3(eta_3, gamma_3)

T_Fb_FA = [cos(eta_3),0,-sin(eta_3) ;...
            sin(eta_3)*sin(gamma_3),cos(gamma_3),cos(eta_3)*sin(gamma_3);...
            sin(eta_3)*cos(gamma_3),-sin(gamma_3),cos(eta_3)*cos(gamma_3)];

== matlab function Trim_Model/3 Copter Complete/Arms Dynamics: Forces and Moments/Arm 2 Dynamics/Arms Kinematics/DCM Arm 2 ==
  data: eta_2 input; T_Fb_FA output; gamma_2 input
function T_Fb_FA = DCM_Arm_2(eta_2, gamma_2)

T_Fb_FA = [cos(eta_2),0,-sin(eta_2) ;...
            sin(eta_2)*sin(gamma_2),cos(gamma_2),cos(eta_2)*sin(gamma_2);...
            sin(eta_2)*cos(gamma_2),-sin(gamma_2),cos(eta_2)*cos(gamma_2)];
